simulink model "Delta_Omega_Based_Arduino_TCS"  (R2021a)
settings: Solver=FixedStepAuto  StartTime=0.0  StopTime=100  FixedStep=0.001  RelTol=1e-3  EnableMultiTasking=on
values from neighbouring files (symbols this model uses):
  GR = 5    [Model_Data.mat]
  grade = 0    [Model_Data.mat]
  m = 220    [Model_Data.mat]
  r = 0.3059    [Model_Data.mat]
  s2_5_rps = [0 104.6666667 209.3333333 314 418.6666667 523.3333333 628]    [Model_Data.mat]
  s2_5_trq = [70 65 60 50 40 33 27]    [Model_Data.mat]
undefined symbols (not defined in the file or in its folder): conv, h, km, s, T, w
libraries: autolibshared x4, autolibmappedmotor x2, simulink x2, aerolibconvert2 x2, arduinolib x1
(part 3 of 3)

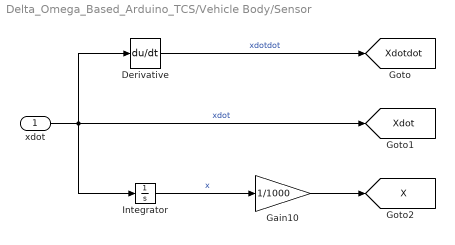
== system Delta_Omega_Based_Arduino_TCS/Vehicle Body/Sensor ==
  xdot : Inport
  Derivative : Derivative
  Gain10 : Gain  Gain=1/1000
  Integrator : Integrator
  tag scope: X=global, Xdot=global, Xdotdot=global
  wires:
  Integrator/1 -> Gain10/1  "x"
  Gain10/1 -> [X]
  xdot/1 -> [Xdot], Integrator/1, Derivative/1  "xdot"
  Derivative/1 -> [Xdotdot]  "xdotdot"

== matlab function Delta_Omega_Based_Arduino_TCS/Traction Controller ==
  data: Difference input; acc_out output; Driver_Command input; velocity input
function acc_out  = fcn(Difference,Driver_Command,velocity)
if (velocity < 1.38)                % Velocity is passed as m/s. 5 km/hr = 1.38 m/s
    if (Difference<0.03)
    acc_out = Driver_Command;
    elseif (Difference>0.03 && Difference<0.05)
    acc_out = 0.8*Driver_Command;
    elseif (Difference>0.05 && Difference<0.2)
    acc_out = 0.6*Driver_Command;
    elseif (Difference>0.2)
    acc_out = 0.4*Driver_Command;
    else
    acc_out = Driver_Command;
    end
%elseif (velocity >= 5)
    %acc_out = Driver_Command;
else
    acc_out = Driver_Command;
            
 end

== matlab function Delta_Omega_Based_Arduino_TCS/OIOO Subsystem1/MATLAB Function ==
  data: u input; y output; mode input
function y = fcn(u, mode)

if mode == 1
    y = 0.8*(u^2);
elseif mode == 2
    y = 0.9*u;
elseif mode == 3
    y = (abs(u)^0.5);
else
    y = 0;
end
